simulink library "rotationAboutX"  (R2020a)
settings: Solver=VariableStepAuto  StartTime=0.0  StopTime=10.0  RelTol=1e-3
libraries: sharedutil x1
settings Model: Creator=Ayaz  LastModifiedBy=Ayaz

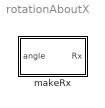
== system rotationAboutX ==
  makeRx : Subsystem

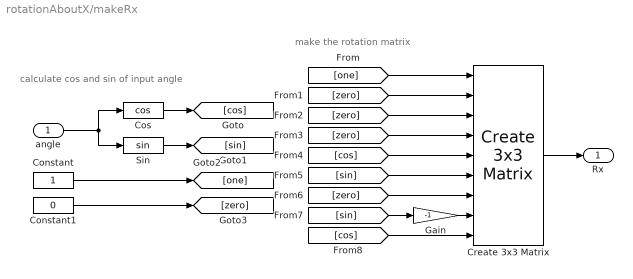
== system rotationAboutX/makeRx ==
  note: make the rotation matrix
  note: calculate cos and sin of input angle
  angle : Inport
  Constant : Constant  VectorParams1D=off
  Constant1 : Constant  Value=0  VectorParams1D=off
  Cos : Trigonometry  Operator=cos
  Create 3x3 Matrix : sharedutil/Create 3x3 Matrix  aMode=aMode
      settings: SourceProductBaseCode=AE,PW,MT,VE,VP
  Gain : Gain  Gain=-1
  Sin : Trigonometry
  Rx : Outport
  wires:
  angle/1 -> Sin/1, Cos/1
  Cos/1 -> [cos]
  Sin/1 -> [sin]
  Constant/1 -> [one]
  Constant1/1 -> [zero]
  [one] -> Create 3x3 Matrix/1
  [zero] -> Create 3x3 Matrix/2
  [zero] -> Create 3x3 Matrix/3
  [zero] -> Create 3x3 Matrix/4
  [cos] -> Create 3x3 Matrix/5
  [sin] -> Create 3x3 Matrix/6
  [zero] -> Create 3x3 Matrix/7
  [sin] -> Gain/1
  Gain/1 -> Create 3x3 Matrix/8
  [cos] -> Create 3x3 Matrix/9
  Create 3x3 Matrix/1 -> Rx/1
